simulink model "Excavator_Mevea_Bucket"  (R2026a)
settings: Solver=ode23t  StopTime=stopTime  FixedStep=1e-5  MaxStep=Ts  AbsTol=1e-3
PostLoadFcn:
  | set_param(bdroot,'IgnoredZcDiagnostic','none');
  | Excavator_Test_Scenario_Select('loadedBucketDigCycle');
  | Excavator_Mevea_params
StartFcn:
  | tStart = tic;
StopFcn:
  | elapsedSimTime = toc(tStart);
  | disp(['Elapsed Sim Time = ' num2str(elapsedSimTime)]);
model workspace: external: MAT-File ExcavatorAssemblyDataStruct.mat (data not in the file)
undefined symbols (not defined in the file or in its folder): AToBRegOrificeVector, AToTOrificeVector, BiPOrificeVector, BoomC, boomHEArea, boomREArea, boomUpMaxQ, boomValve, BToTOrificeVector, BucketC, bucketCloseMaxQ, bucketOpenMaxQ, BucketR, bucketValve, fluids, gravity, LeftBoomR, maxPumpDisp, minPumpDisp, nominalEngineSpeed, P28Assembly, PToAOrificeVector, PToBOrificeVector, pumpCmdNegRateLimit, pumpCmdPosRateLimit, RightBoomR, StickC, stickInMaxQ, stickOutMaxQ, StickR, stickValve, SwingC, swingDisplacement, swingHighSpeedThreshold, swingMaxQ, SwingR, swingSpeedQGain, swingValve, valveCmdNegRateLimit, valveCmdPosRateLimit, X, Y, Z
libraries: fl_lib x89, sm_lib x79, SimscapeFluids_lib x78, nesl_utility x57, simulink_extras x11, Excavator_Parts_Lib x6, SignalEditorBlockLib x1
(part 1 of 7)
Description:
  | Copyright 2022-2026 The MathWorks, Inc.
settings Model: VariantFading=off  Creator=gabri  LastModifiedBy=smiller
settings SolverCC: MaxConsecutiveMinStep=10  ZeroCrossAlgorithm=Adaptive  DecoupledContinuousIntegration=on  MinimalZcImpactIntegration=on
settings DataIOCC: ExternalInput=activeTestCmdsMevea  LoadExternalInput=on  SignalLoggingName=logsout_Excavator_Complete  OutputTimes=[0:Ts:stopTime]  ReturnWorkspaceOutputsName=simOut
settings DebuggingCC: IgnoredZcDiagnostic=none
settings SimscapeCC: SimscapeNominalValues="[{\"value\":\"1\",\"unit\":\"A\"},{\"value\":\"1\",\"unit\":\"bar\"},{\"value\":\"1\",\"unit\":\"cm^2\"},{\"value\":\"1\",\"unit\":\"cm^3/s\"},{\"value\":\"1\",\"unit\":\"kJ/kg\"},{\"value\":\"1\",\"unit\":\"kW\"},{\"value\":\"1\",\"unit\":\"l\"},{\"value\":\"1\",\"unit\":\"N\"},{\"value\":\"1\",\"unit\":\"N*m\"},{\"value\":\"1\",\"unit\":\"V\"}]"  SimscapeLogName=simlog_Excavator_Complete  SimscapeLogLimitData=off  SimscapeLogDataHistory=5000.0
settings DiagnosticsConfigSet: SimMechanicsUnconnectedFramePorts=none  SimMechanicsConflictingReferenceFrames=none
settings ExplorerConfigSet: InternalSimMechanicsExplorerSettings="<ExplorerConfiguration><canonicalview>default</canonicalview><AnimationSetting><BasePlaybackSpeed>1.0</BasePlaybackSpeed><PlaybackSpeedFactor>1.0</PlaybackSpeedFactor></AnimationSetting><TilePanel><TileInfo><Tiles Columns=\"1\" Count=\"1\" Rows=\"1\"><Column Weight=\"1\"/><Row Weight=\"1\"/><Tile Height=\"1\" Width=\"1\" X=\"0\" Y=\"0\"/></Tiles></TileInfo><SceneInfo><SceneViewer><BGColor><R>1</R><G>1</G><B>1</B></BGColor><Camera><DoPerspective>off</DoPerspective><Position><X>63.5460374940453718</X><Y>-11.8017502462116433</Y><Z>6.23155607724029448</Z></Position><Center><X>32.4989157916715854</X><Y>-5.03969608578851869</Y><Z>4.87768395327128346</Z></Center><Up><X>-0.0494260662251312932</X><Y>-0.0270354491512150297</Y><Z>0.998411813064479459</Z></Up><ViewLimDist>1</ViewLimDist><YLim>6.89330450435498676</YLim><XLim>8.26192051705934638</XLim></Camera></SceneViewer></SceneInfo></TilePanel><MechEditorPanel><Cameras/><GfxPanelCameraMap/><VideoCreator><PlaybackSpeedRatio>1.0</PlaybackSpeedRatio><FrameRate>30</FrameRate><VideoFormat>Motion JPEG AVI</VideoFormat><FrameSize>auto</FrameSize></VideoCreator></MechEditorPanel></ExplorerConfiguration>"

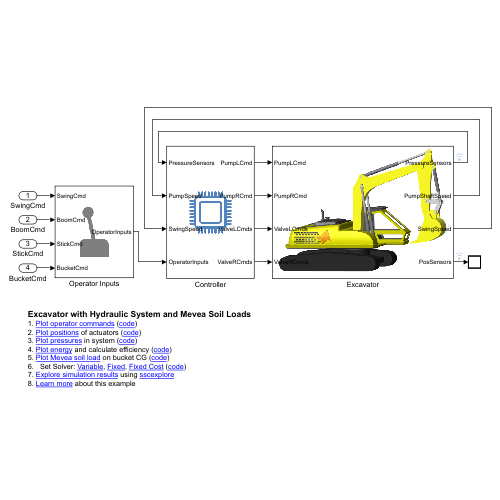
[thumbnail: Simulink's stored preview of the top-level diagram]
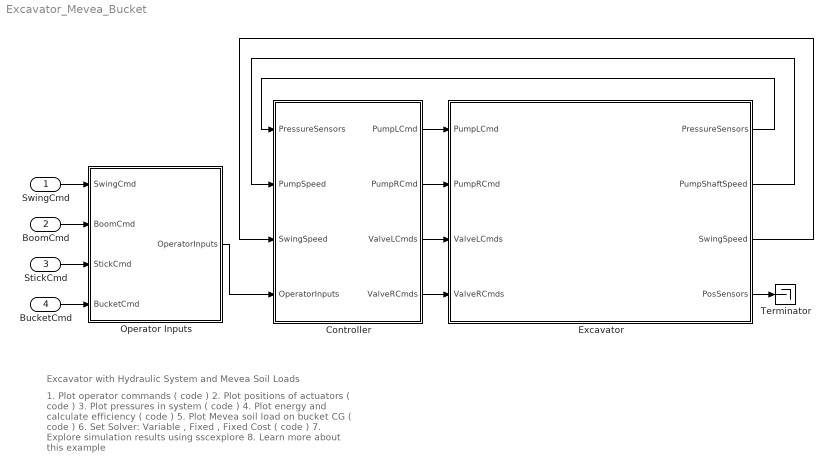
== system Excavator_Mevea_Bucket ==
  note: Excavator with Hydraulic System and Mevea Soil Loads
  note: 1. Plot operator commands ( code )
      | 2. Plot positions of actuators ( code )
      | 3. Plot pressures in system ( code )
      | 4. Plot energy and calculate efficiency ( code )
      | 5. Plot Mevea soil load on bucket CG ( code )
      | 6. Set Solver: Variable , Fixed , Fixed Cost ( code )
      | 7. Explore simulation results using sscexplore
      | 8. Learn more about this example
  SwingCmd : Inport
  BoomCmd : Inport  Port=2
  StickCmd : Inport  Port=3
  BucketCmd : Inport  Port=4
  Controller : Subsystem
      mask Display: image('Excavator_Controller_IMAGE.png')
  Excavator : Subsystem
      mask Display: image('Excavator_CAD_Full_IMAGE.png');
  Operator Inputs : Subsystem
      mask Display: image('Excavator_Operator_Inputs_IMAGE.png')
  Terminator : Terminator
  wires:
  Excavator/2(PumpShaftSpeed) -> Controller/2(PumpSpeed)
  Controller/3(ValveLCmds) -> Excavator/3(ValveLCmds)
  Operator Inputs/1(OperatorInputs) -> Controller/4(OperatorInputs)
  Excavator/1(PressureSensors) -> Controller/1(PressureSensors)
  Controller/4(ValveRCmds) -> Excavator/4(ValveRCmds)
  Controller/1(PumpLCmd) -> Excavator/1(PumpLCmd)
  Controller/2(PumpRCmd) -> Excavator/2(PumpRCmd)
  SwingCmd/1 -> Operator Inputs/1(SwingCmd)
  BoomCmd/1 -> Operator Inputs/2(BoomCmd)
  StickCmd/1 -> Operator Inputs/3(StickCmd)
  BucketCmd/1 -> Operator Inputs/4(BucketCmd)
  Excavator/3(SwingSpeed) -> Controller/3(SwingSpeed)
  Excavator/4(PosSensors) -> Terminator/1

== system Excavator_Mevea_Bucket/Controller ==
  PressureSensors : Inport
  PumpSpeed : Inport  Port=2
  SwingSpeed : Inport  Port=3
  OperatorInputs : Inport  Port=4
  Function Commander : Subsystem
  PumpLCmd : Outport
  PumpRCmd : Outport  Port=2
  ValveLCmds : Outport  Port=3
  ValveRCmds : Outport  Port=4
  wires:
  Function Commander/1(PumpLCmd) -> PumpLCmd/1
  Function Commander/3(LeftValveCmds) -> ValveLCmds/1
  Function Commander/2(PumpRCmd) -> PumpRCmd/1
  Function Commander/4(RightValveCmds) -> ValveRCmds/1
  PressureSensors/1 -> Function Commander/2(PressureSensors)
  OperatorInputs/1 -> Function Commander/1(OperatorInputs)
  PumpSpeed/1 -> Function Commander/3(PumpSpeed)
  SwingSpeed/1 -> Function Commander/4(SwingSpeed)

== system Excavator_Mevea_Bucket/Excavator ==
  PumpLCmd : Inport
  PumpRCmd : Inport  Port=2
  ValveLCmds : Inport  Port=3
  ValveRCmds : Inport  Port=4
  Engine : Subsystem
      settings: PortSchema="{\"entries\":[{\"content\":{\"sides\":[{\"content\":{\"connectorIds\":[]},\"type\":\"ConnectorPlacement.EquallySpacedRectSide\",\"uuid\":\"32d181a9-9647-459e-8a6e-f34844cbb584\"},{\"content\":{\"connectorIds\":[\"RConn1\",\"Out1\"],\"side\":\"RIGHT\"},\"type\":\"ConnectorPlacement.EquallySpacedRectSide\",\"uuid\":\"3f25e2ea-f411-44b7-ab9d-c86c977187b2\"},{\"content\":{\"connectorIds\":[],\"side\":\"TOP\"},\"type\":\"ConnectorPlacement.EquallySpacedRectSide\",\"uuid\":\"8da3c69e-7eb0-422f-a85f-a16d195e09d7\"}]},\"type\":\"ConnectorPlacement.EquallySpacedConnector\",\"uuid\":\"c91a59d7-4912-461c-aac6-1d25f9b3f709\"}],\"packageUris\":[\"http://schema.mathworks.com/mf0/Connector/R2020b\"],\"version\":\"1.0\"}"
      mask Display: image('Engine_IMAGE.png')
  Hydraulics : Subsystem
      mask Display: image('Hydraulic_System_IMAGE.png');
  Machine : Subsystem
      mask Display: image('Excavator_CAD_Full_IMAGE.png');
  PressureSensors : Outport
  PumpShaftSpeed : Outport  Port=2
  SwingSpeed : Outport  Port=3
  PosSensors : Outport  Port=4
  wires:
  Engine/1(PumpShaftSpeed) -> PumpShaftSpeed/1
  PumpLCmd/1 -> Hydraulics/1(PumpLCmd)
  PumpRCmd/1 -> Hydraulics/2(PumpRCmd)
  ValveLCmds/1 -> Hydraulics/3(ValveLCmds)
  ValveRCmds/1 -> Hydraulics/4(ValveRCmds)
  Hydraulics/1(mPr) -> PressureSensors/1
  Machine/1(SwingSpeed) -> SwingSpeed/1
  Hydraulics/2(mPos) -> PosSensors/1
  connections:
  Hydraulics/RConn1 -- Machine/LConn1
  Hydraulics/RConn2 -- Machine/LConn2
  Hydraulics/RConn3 -- Machine/LConn3
  Hydraulics/RConn4 -- Machine/LConn4
  Engine/RConn1 -- Hydraulics/LConn1

== system Excavator_Mevea_Bucket/Operator Inputs ==
  note: This Signal Editor block is here to allow for manipulation of the
      | dig cycle commands. The single function tests use the 'TestCmds'
      | scenario which is modified programatically for the function to be
      | tested when the 'TestScenarioDefinitions' script is ran.
      |
      | The inports at the top level of the model bring the commands in for
      | the simulation and are put into a bus here.
  SwingCmd : Inport
  BoomCmd : Inport  Port=2
  StickCmd : Inport  Port=3
  BucketCmd : Inport  Port=4
  OpCmdBusCreator : BusCreator  Inputs=4
  Signal Editor : SignalEditorBlockLib/Signal Editor  Commented=on  FileName=TestCommands.mat  ActiveScenario=TestCmds  ActiveSignal=SwingCmd  IsBus=off  OutputBusObjectStr=Bus: BusObject  SampleTime=0  Interpolate=off  ZeroCross=off  OutputAfterFinalValue=Setting to zero  Unit=inherit  PreserveSignalName=on  ApplySigPropsToAllScenarios=on  ApplySigPropsToAllSignals=off  SignalPropertySource=Dialog parameters
  OperatorInputs : Outport
  wires:
  OpCmdBusCreator/1 -> OperatorInputs/1
  SwingCmd/1 -> OpCmdBusCreator/1  "swingCmd"
  BoomCmd/1 -> OpCmdBusCreator/2  "boomCmd"
  StickCmd/1 -> OpCmdBusCreator/3  "stickCmd"
  BucketCmd/1 -> OpCmdBusCreator/4  "bucketCmd"

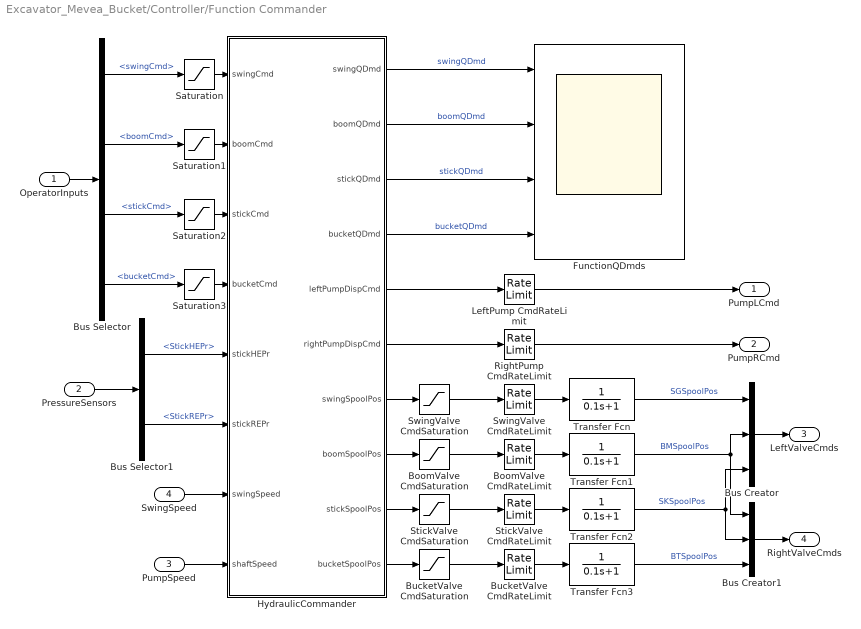
== system Excavator_Mevea_Bucket/Controller/Function Commander ==
  OperatorInputs : Inport
  PressureSensors : Inport  Port=2
  PumpSpeed : Inport  Port=3
  SwingSpeed : Inport  Port=4
  BoomValve CmdRateLimit : RateLimiter  RisingSlewLimit=valveCmdPosRateLimit  FallingSlewLimit=valveCmdNegRateLimit  SampleTimeMode=inherited
  BoomValve CmdSaturation : Saturate  UpperLimit=5  LowerLimit=-5  ZeroCross=off
  BucketValve CmdRateLimit : RateLimiter  RisingSlewLimit=valveCmdPosRateLimit  FallingSlewLimit=valveCmdNegRateLimit  SampleTimeMode=inherited
  BucketValve CmdSaturation : Saturate  UpperLimit=5  LowerLimit=-5  ZeroCross=off
  Bus Creator : BusCreator  Inputs=3
  Bus Creator1 : BusCreator  Inputs=3
  Bus Selector : BusSelector  OutputSignals=swingCmd,boomCmd,stickCmd,bucketCmd
  Bus Selector1 : BusSelector  OutputSignals=StickHEPr,StickREPr
  FunctionQDmds : Scope  NumInputPorts=4
      settings: ActiveDisplayYMinimum=-87.5  ActiveDisplayYMaximum=787.5
  HydraulicCommander : MATLAB Function  TreatAsAtomicUnit=on  mask{swingMaxQ=swingMaxQ, boomUpMaxQ=boomUpMaxQ, stickInMaxQ=stickInMaxQ, stickOutMaxQ=stickOutMaxQ, bucketOpenMaxQ=bucketOpenMaxQ, bucketCloseMaxQ=bucketCloseMaxQ, nominalShaftSpeed=nominalEngineSpeed, minPumpDisp=minPumpDisp, maxPumpDisp=maxPumpDisp, swingSpeedQGain=swingSpeedQGain, swingHighSpeedThreshold=swingHighSpeedThreshold}
      mask prompts: swingMaxQ "Swing Max Flow Rate [lpm]:"; boomUpMaxQ "Boom Up Max Flow Rate [lpm]:"; stickInMaxQ "Stick In Max Flow Rate [lpm]:"; stickOutMaxQ "Stick Out Max Flow Rate [lpm]:"; bucketOpenMaxQ "Bucket Open Max Flow Rate [lpm]:"; bucketCloseMaxQ "Bucket Close Max Flow Rate [lpm]:"; nominalShaftSpeed "Nominal Shaft Speed [rpm]:"; minPumpDisp "Minimum Pump Displacement [cc/rev]:"; maxPumpDisp "Maximum Pump Displacement [cc/rev]:"; swingSpeedQGain "Swing Flow Rate Optimization Gain:"; swingHighSpeedThreshold "Swing High Speed Threshold [rpm]:"
  LeftPump CmdRateLimit : RateLimiter  RisingSlewLimit=pumpCmdPosRateLimit  FallingSlewLimit=pumpCmdNegRateLimit  SampleTimeMode=inherited
  RightPump CmdRateLimit : RateLimiter  RisingSlewLimit=pumpCmdPosRateLimit  FallingSlewLimit=pumpCmdNegRateLimit  SampleTimeMode=inherited
  Saturation{,1..3} (4 alike) : Saturate  UpperLimit=1  LowerLimit=-1  ZeroCross=off
  StickValve CmdRateLimit : RateLimiter  RisingSlewLimit=valveCmdPosRateLimit  FallingSlewLimit=valveCmdNegRateLimit  SampleTimeMode=inherited
  StickValve CmdSaturation : Saturate  UpperLimit=5  LowerLimit=-5  ZeroCross=off
  SwingValve CmdRateLimit : RateLimiter  RisingSlewLimit=valveCmdPosRateLimit  FallingSlewLimit=valveCmdNegRateLimit  SampleTimeMode=inherited
  SwingValve CmdSaturation : Saturate  UpperLimit=5  LowerLimit=-5  ZeroCross=off
  Transfer Fcn{,1..3} (4 alike) : TransferFcn  Denominator=[0.1 1]
  PumpLCmd : Outport
  PumpRCmd : Outport  Port=2
  LeftValveCmds : Outport  Port=3
  RightValveCmds : Outport  Port=4
  wires:
  OperatorInputs/1 -> Bus Selector/1
  Bus Selector/4 -> Saturation3/1  "<bucketCmd>"
  Bus Selector/3 -> Saturation2/1  "<stickCmd>"
  Bus Selector/2 -> Saturation1/1  "<boomCmd>"
  Bus Selector/1 -> Saturation/1  "<swingCmd>"
  PumpSpeed/1 -> HydraulicCommander/8(shaftSpeed)
  PressureSensors/1 -> Bus Selector1/1
  Bus Selector1/1 -> HydraulicCommander/5(stickHEPr)  "<StickHEPr>"
  Bus Selector1/2 -> HydraulicCommander/6(stickREPr)  "<StickREPr>"
  Bus Creator/1 -> LeftValveCmds/1
  Bus Creator1/1 -> RightValveCmds/1
  HydraulicCommander/1(swingQDmd) -> FunctionQDmds/1  "swingQDmd"
  HydraulicCommander/2(boomQDmd) -> FunctionQDmds/2  "boomQDmd"
  HydraulicCommander/3(stickQDmd) -> FunctionQDmds/3  "stickQDmd"
  HydraulicCommander/4(bucketQDmd) -> FunctionQDmds/4  "bucketQDmd"
  Transfer Fcn1/1 -> Bus Creator1/1, Bus Creator/2  "BMSpoolPos"
  Transfer Fcn/1 -> Bus Creator/1  "SGSpoolPos"
  Transfer Fcn2/1 -> Bus Creator1/2, Bus Creator/3  "SKSpoolPos"
  Transfer Fcn3/1 -> Bus Creator1/3  "BTSpoolPos"
  LeftPump CmdRateLimit/1 -> PumpLCmd/1
  RightPump CmdRateLimit/1 -> PumpRCmd/1
  Saturation/1 -> HydraulicCommander/1(swingCmd)
  Saturation1/1 -> HydraulicCommander/2(boomCmd)
  Saturation2/1 -> HydraulicCommander/3(stickCmd)
  Saturation3/1 -> HydraulicCommander/4(bucketCmd)
  SwingSpeed/1 -> HydraulicCommander/7(swingSpeed)
  SwingValve CmdSaturation/1 -> SwingValve CmdRateLimit/1
  BoomValve CmdSaturation/1 -> BoomValve CmdRateLimit/1
  StickValve CmdSaturation/1 -> StickValve CmdRateLimit/1
  BucketValve CmdSaturation/1 -> BucketValve CmdRateLimit/1
  HydraulicCommander/5(leftPumpDispCmd) -> LeftPump CmdRateLimit/1
  HydraulicCommander/6(rightPumpDispCmd) -> RightPump CmdRateLimit/1
  HydraulicCommander/7(swingSpoolPos) -> SwingValve CmdSaturation/1
  HydraulicCommander/8(boomSpoolPos) -> BoomValve CmdSaturation/1
  HydraulicCommander/9(stickSpoolPos) -> StickValve CmdSaturation/1
  HydraulicCommander/10(bucketSpoolPos) -> BucketValve CmdSaturation/1
  SwingValve CmdRateLimit/1 -> Transfer Fcn/1
  BoomValve CmdRateLimit/1 -> Transfer Fcn1/1
  StickValve CmdRateLimit/1 -> Transfer Fcn2/1
  BucketValve CmdRateLimit/1 -> Transfer Fcn3/1

== system Excavator_Mevea_Bucket/Excavator/Engine ==
  Engine : fl_lib/Mechanical/Mechanical Sources/Ideal Angular Velocity Source
  EngineRotationalRef : fl_lib/Mechanical/Rotational Elements/Mechanical Rotational Reference
  Ideal Rotational Motion Sensor : fl_lib/Mechanical/Mechanical Sensors/Ideal Rotational Motion Sensor  reference=foundation.enum.MeasurementReference.difference  acceleration_port=false  velocity_port=true  position_port=true  wrap_angle=simscape.enum.onoff.off  offset=0 rad
  PS Constant : fl_lib/Physical Signals/Sources/PS Constant  constant=1500 rpm
  PS-Simulink Converter : nesl_utility/PS-Simulink Converter  PhysicalDomain=network_engine_domain  SubClassName=ps_output  LeftPortType=input  RightPortType=output  PseudoPeriodic=off  Frequencies=[]  VectorFormat=1-D array  Unit=rpm  AffineConversion=off
  PS-Simulink Converter3 : nesl_utility/PS-Simulink Converter  PhysicalDomain=network_engine_domain  SubClassName=ps_output  LeftPortType=input  RightPortType=output  PseudoPeriodic=off  Frequencies=[]  VectorFormat=1-D array  Unit=rad  AffineConversion=off
  Terminator : Terminator
  Transfer Fcn (with initial outputs) : simulink_extras/Additional Linear/Transfer Fcn (with initial outputs)  N=[1]  D="[0.01  1]"  Y0=1500  U0=1500
  Shaft : PMIOPort  Side=Right
  PumpShaftSpeed : Outport
  wires:
  PS-Simulink Converter/1 -> Transfer Fcn (with initial outputs)/1
  PS-Simulink Converter3/1 -> Terminator/1
  Transfer Fcn (with initial outputs)/1 -> PumpShaftSpeed/1
  connections:
  PS Constant/RConn1 -- Engine/RConn1
  Engine/RConn2 -- Ideal Rotational Motion Sensor/RConn1 -- EngineRotationalRef/LConn1
  Shaft/RConn1 -- Ideal Rotational Motion Sensor/LConn1 -- Engine/LConn1
  PS-Simulink Converter3/LConn1 -- Ideal Rotational Motion Sensor/RConn3
  Ideal Rotational Motion Sensor/RConn2 -- PS-Simulink Converter/LConn1

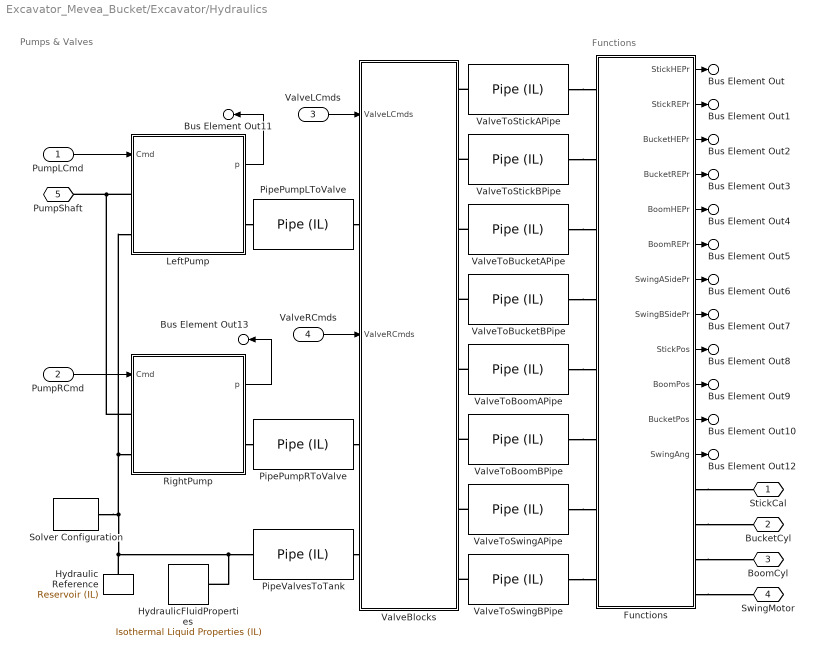
== system Excavator_Mevea_Bucket/Excavator/Hydraulics ==
  note: Functions
  note: Pumps & Valves
  PumpLCmd : Inport
  PumpRCmd : Inport  Port=2
  ValveLCmds : Inport  Port=3
  ValveRCmds : Inport  Port=4
  Functions : Subsystem
      mask Display: image('Hydraulic_Actuators_All_IMAGE.png');
  Hydraulic Reference : fl_lib/Isothermal Liquid/Elements/Reservoir (IL)  pressure_input=false  pressure_spec=foundation.enum.pressure_spec.atmospheric  reservoir_pressure=0.101325 MPa
  HydraulicFluidProperties : fl_lib/Isothermal Liquid/Utilities/Isothermal Liquid Properties (IL)  rho_L_atm=870 kg/m^3  bulk_modulus_model=foundation.enum.bulk_modulus_model.const  beta_gain=6  beta_L_atm=1.45e9 Pa  nu_atm=46 mm^2/s  p_atm=0.101325 MPa  p_min=0.1 Pa  properties_range_check=simscape.enum.assert.action.error  air_fraction=0.005  polytropic_index=1.0  rho_g_atm=1.225 kg/m^3  air_dissolution_model=simscape.enum.onoff.off  p_crit=3 MPa
  LeftPump : Subsystem
      mask Display: image('Hydraulic_Pump_IMAGE.png')
  PipePumpLToValve : fl_lib/Isothermal Liquid/Elements/Pipe (IL)  length=pipeLength mm  area=pipeCrossSectArea mm^2  Dh=pipeHydraulicDiam mm  length_add=1 m  roughness=15e-6 m  Re_lam=2000  Re_tur=4000  shape_factor=64  dynamic_compressibility=simscape.enum.onoff.off  inertia=simscape.enum.onoff.off  p0=0.101325 MPa  mdot0=0 kg/s
  PipePumpRToValve : fl_lib/Isothermal Liquid/Elements/Pipe (IL)  length=pipeLength mm  area=pipeCrossSectArea mm^2  Dh=pipeHydraulicDiam mm  length_add=1 m  roughness=15e-6 m  Re_lam=2000  Re_tur=4000  shape_factor=64  dynamic_compressibility=simscape.enum.onoff.off  inertia=simscape.enum.onoff.off  p0=0.101325 MPa  mdot0=0 kg/s
  PipeValvesToTank : fl_lib/Isothermal Liquid/Elements/Pipe (IL)  length=pipeLength mm  area=pipeCrossSectArea mm^2  Dh=pipeHydraulicDiam mm  length_add=1 m  roughness=15e-6 m  Re_lam=2000  Re_tur=4000  shape_factor=64  dynamic_compressibility=simscape.enum.onoff.off  inertia=simscape.enum.onoff.off  p0=0.101325 MPa  mdot0=0 kg/s
  RightPump : Subsystem
      mask Display: image('Hydraulic_Pump_IMAGE.png')
  Solver Configuration : nesl_utility/Solver Configuration  PhysicalDomain=network_engine_domain  SubClassName=solver  LeftPortType=input  RightPortType=generic  Tones=[]  Harmonics=[]  SimulateNoise=off  Profile=off  UseLocalSampling=off  EnableSwitchedLinearOptims=on  FrequencyDomain=off  UseCCode=off  RelTol=0.001  AbsTol=1e-06  MinStep=1e-09  ToWorkspace=off  RevertToSquareIcSolve=off  NumHomotopyIterations=100  PhasorMode=off  PhasorModeNumHarmonics=1  ConsistencySolver=NEWTON_FTOL  CanonicalOrdering=UNORDERED  OptimizeIntermediates=UNOPTIMIZED  IndexReductionMethod=DerivativeReplacement  DoDC=off  ResidualTolerance=1e-09  ConsistencyTolSource=GLOBAL  ConsistencyAbsTol=0.001  ConsistencyRelTol=0.001  ConsistencyTolFactor=0.001  UseLocalSolver=off  LocalSolverChoice=NE_BACKWARD_EULER_ADVANCER  ResolveIndetEquations=on  FunctionEvalNumThread=1  LocalSolverSampleTime=0.001  DoFixedCost=off  MaxNonlinIter=3  MaxModeIter=2  ComputeImpulses=off  ImpulseIterations=2  LinearAlgebra=auto  LinearAlgebraNumThread=0  EquationFormulation=NE_TIME_EF  DelaysMemoryBudget=1024  AutomaticFiltering=on  FilteringTimeConstant=0.001  PartitionStorageMethod=AS_NEEDED  PartitionMemoryBudget=1024  PartitionMethod=ROBUST  MultibodyUseLocalSolver=off  MultibodyLocalSolverChoice=ODE1  MultibodyLocalSolverSampleTime=0.001
  ValveBlocks : Subsystem
      settings: PortSchema="{\"entries\":[{\"content\":{\"sides\":[{\"content\":{\"connectorIds\":[\"In1\",\"LConn1\",\"In2\",\"LConn2\",\"LConn3\"]},\"type\":\"ConnectorPlacement.EquallySpacedRectSide\",\"uuid\":\"b3bc2bda-0212-4e11-9874-ac6e4fe9b6a3\"},{\"content\":{\"connectorIds\":[\"RConn1\",\"RConn2\",\"RConn3\",\"RConn4\",\"RConn5\",\"RConn6\",\"RConn7\",\"RConn8\"],\"side\":\"RIGHT\"},\"type\":\"ConnectorPlacement.EquallySpacedRectSide\",\"uuid\":\"c9983e91-7586-4f39-92a2-b2598f03e211\"},{\"content\":{\"connectorIds\":[],\"side\":\"TOP\"},\"type\":\"ConnectorPlacement.EquallySpacedRectSide\",\"uuid\":\"d3f67102-423e-42f5-ac92-8a3282aefd24\"}]},\"type\":\"ConnectorPlacement.EquallySpacedConnector\",\"uuid\":\"bd5efcea-2b0a-45c5-b20e-e10c208a7bb5\"}],\"packageUris\":[\"http://schema.mathworks.com/mf0/Connector/R2020b\"],\"version\":\"1.0\"}"
      mask Display: image('Valve_Block_All_IMAGE.png')
  ValveToBoomAPipe : fl_lib/Isothermal Liquid/Elements/Pipe (IL)  length=pipeLength mm  area=pipeCrossSectArea mm^2  Dh=pipeHydraulicDiam mm  length_add=1 m  roughness=15e-6 m  Re_lam=2000  Re_tur=4000  shape_factor=64  dynamic_compressibility=simscape.enum.onoff.off  inertia=simscape.enum.onoff.off  p0=0.101325 MPa  mdot0=0 kg/s
  ValveToBoomBPipe : fl_lib/Isothermal Liquid/Elements/Pipe (IL)  length=pipeLength mm  area=pipeCrossSectArea mm^2  Dh=pipeHydraulicDiam mm  length_add=1 m  roughness=15e-6 m  Re_lam=2000  Re_tur=4000  shape_factor=64  dynamic_compressibility=simscape.enum.onoff.off  inertia=simscape.enum.onoff.off  p0=0.101325 MPa  mdot0=0 kg/s
  ValveToBucketAPipe : fl_lib/Isothermal Liquid/Elements/Pipe (IL)  length=pipeLength mm  area=pipeCrossSectArea mm^2  Dh=pipeHydraulicDiam mm  length_add=1 m  roughness=15e-6 m  Re_lam=2000  Re_tur=4000  shape_factor=64  dynamic_compressibility=simscape.enum.onoff.off  inertia=simscape.enum.onoff.off  p0=0.101325 MPa  mdot0=0 kg/s
  ValveToBucketBPipe : fl_lib/Isothermal Liquid/Elements/Pipe (IL)  length=pipeLength mm  area=pipeCrossSectArea mm^2  Dh=pipeHydraulicDiam mm  length_add=1 m  roughness=15e-6 m  Re_lam=2000  Re_tur=4000  shape_factor=64  dynamic_compressibility=simscape.enum.onoff.off  inertia=simscape.enum.onoff.off  p0=0.101325 MPa  mdot0=0 kg/s
  ValveToStickAPipe : fl_lib/Isothermal Liquid/Elements/Pipe (IL)  length=pipeLength mm  area=pipeCrossSectArea mm^2  Dh=pipeHydraulicDiam mm  length_add=1 m  roughness=15e-6 m  Re_lam=2000  Re_tur=4000  shape_factor=64  dynamic_compressibility=simscape.enum.onoff.off  inertia=simscape.enum.onoff.off  p0=0.101325 MPa  mdot0=0 kg/s
  ValveToStickBPipe : fl_lib/Isothermal Liquid/Elements/Pipe (IL)  length=pipeLength mm  area=pipeCrossSectArea mm^2  Dh=pipeHydraulicDiam mm  length_add=1 m  roughness=15e-6 m  Re_lam=2000  Re_tur=4000  shape_factor=64  dynamic_compressibility=simscape.enum.onoff.off  inertia=simscape.enum.onoff.off  p0=0.101325 MPa  mdot0=0 kg/s
  ValveToSwingAPipe : fl_lib/Isothermal Liquid/Elements/Pipe (IL)  length=pipeLength mm  area=pipeCrossSectArea mm^2  Dh=pipeHydraulicDiam mm  length_add=1 m  roughness=15e-6 m  Re_lam=2000  Re_tur=4000  shape_factor=64  dynamic_compressibility=false  inertia=simscape.enum.onoff.off  p0=initSwingAPr MPa  mdot0=0 kg/s
  ValveToSwingBPipe : fl_lib/Isothermal Liquid/Elements/Pipe (IL)  length=pipeLength mm  area=pipeCrossSectArea mm^2  Dh=pipeHydraulicDiam mm  length_add=1 m  roughness=15e-6 m  Re_lam=2000  Re_tur=4000  shape_factor=64  dynamic_compressibility=false  inertia=simscape.enum.onoff.off  p0=initSwingAPr MPa  mdot0=0 kg/s
  StickCal : PMIOPort  Side=Right
  BucketCyl : PMIOPort  Port=2  Side=Right
  BoomCyl : PMIOPort  Port=3  Side=Right
  SwingMotor : PMIOPort  Port=4  Side=Right
  PumpShaft : PMIOPort  Port=5  Side=Left
  Bus Element Out : Outport  PortName=mPr  Element=StickHEPr
  Bus Element Out1 : Outport  PortName=mPr  Element=StickREPr
  Bus Element Out2 : Outport  PortName=mPr  Element=BucketHEPr
  Bus Element Out3 : Outport  PortName=mPr  Element=BucketREPr
  Bus Element Out4 : Outport  PortName=mPr  Element=BoomHEPr
  Bus Element Out5 : Outport  PortName=mPr  Element=BoomREPr
  Bus Element Out6 : Outport  PortName=mPr  Element=SwingASidePr
  Bus Element Out7 : Outport  PortName=mPr  Element=SwingBSidePr
  Bus Element Out11 : Outport  PortName=mPr  Element=LeftPumpPr
  Bus Element Out13 : Outport  PortName=mPr  Element=RightPumpPr
  Bus Element Out12 : Outport  Port=2  PortName=mPos  Element=SwingAng
  Bus Element Out10 : Outport  Port=2  PortName=mPos  Element=BucketPos
  Bus Element Out9 : Outport  Port=2  PortName=mPos  Element=BoomPos
  Bus Element Out8 : Outport  Port=2  PortName=mPos  Element=StickPos
  wires:
  RightPump/1(p) -> Bus Element Out13/1
  PumpLCmd/1 -> LeftPump/1(Cmd)
  LeftPump/1(p) -> Bus Element Out11/1
  ValveRCmds/1 -> ValveBlocks/2(ValveRCmds)
  ValveLCmds/1 -> ValveBlocks/1(ValveLCmds)
  Functions/1(StickHEPr) -> Bus Element Out/1
  Functions/3(BucketHEPr) -> Bus Element Out2/1
  Functions/5(BoomHEPr) -> Bus Element Out4/1
  Functions/7(SwingASidePr) -> Bus Element Out6/1
  Functions/8(SwingBSidePr) -> Bus Element Out7/1
  Functions/6(BoomREPr) -> Bus Element Out5/1
  Functions/4(BucketREPr) -> Bus Element Out3/1
  Functions/2(StickREPr) -> Bus Element Out1/1
  PumpRCmd/1 -> RightPump/1(Cmd)
  Functions/9(StickPos) -> Bus Element Out8/1
  Functions/10(BoomPos) -> Bus Element Out9/1
  Functions/11(BucketPos) -> Bus Element Out10/1
  Functions/12(SwingAng) -> Bus Element Out12/1
  connections:
  LeftPump/LConn1 -- PumpShaft/RConn1 -- RightPump/LConn1
  LeftPump/RConn1 -- PipePumpLToValve/LConn1
  RightPump/RConn1 -- PipePumpRToValve/LConn1
  Functions/RConn1 -- StickCal/RConn1
  Functions/RConn2 -- BucketCyl/RConn1
  Functions/RConn3 -- BoomCyl/RConn1
  Functions/RConn4 -- SwingMotor/RConn1
  PipePumpLToValve/RConn1 -- ValveBlocks/LConn1
  PipePumpRToValve/RConn1 -- ValveBlocks/LConn2
  ValveToStickAPipe/LConn1 -- ValveBlocks/RConn1
  ValveToStickBPipe/LConn1 -- ValveBlocks/RConn2
  ValveToBucketAPipe/LConn1 -- ValveBlocks/RConn3
  ValveToBucketBPipe/LConn1 -- ValveBlocks/RConn4
  ValveToBoomAPipe/LConn1 -- ValveBlocks/RConn5
  ValveToBoomBPipe/LConn1 -- ValveBlocks/RConn6
  ValveToSwingAPipe/LConn1 -- ValveBlocks/RConn7
  ValveToSwingBPipe/LConn1 -- ValveBlocks/RConn8
  ValveToSwingBPipe/RConn1 -- Functions/LConn8
  ValveToSwingAPipe/RConn1 -- Functions/LConn7
  ValveToBoomBPipe/RConn1 -- Functions/LConn6
  ValveToBoomAPipe/RConn1 -- Functions/LConn5
  ValveToBucketBPipe/RConn1 -- Functions/LConn4
  ValveToBucketAPipe/RConn1 -- Functions/LConn3
  ValveToStickBPipe/RConn1 -- Functions/LConn2
  ValveToStickAPipe/RConn1 -- Functions/LConn1
  RightPump/LConn2 -- Hydraulic Reference/LConn1 -- HydraulicFluidProperties/RConn1 -- PipeValvesToTank/RConn1 -- Solver Configuration/RConn1 -- LeftPump/LConn2
  PipeValvesToTank/LConn1 -- ValveBlocks/LConn3

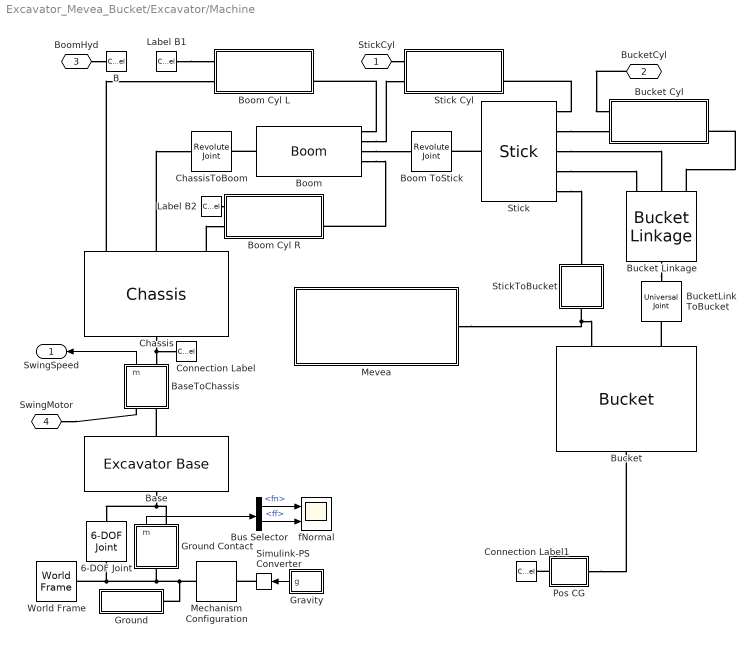
== system Excavator_Mevea_Bucket/Excavator/Machine ==
  6-DOF Joint : sm_lib/Joints/6-DOF Joint  JointMode=Normal  CompositeWrenchDir=FollowerOnBase  CompositeWrenchFrame=BaseFrame  SenseConstraintForce=off  SenseConstraintTorque=off  SenseTotalForce=off  SenseTotalTorque=off  PxPositionTargetSpecify=off  PxPositionTargetPriority=High  PxPositionTargetValue=0  PxPositionTargetValueUnits=m  PxVelocityTargetSpecify=off  PxVelocityTargetPriority=High  PxVelocityTargetValue=0  PxVelocityTargetValueUnits=m/s  PxEquilibriumPosition=0  PxEquilibriumPositionUnits=m  PxSpringStiffness=0  PxSpringStiffnessUnits=N/m  PxDampingCoefficient=0  PxDampingCoefficientUnits=N/(m/s)  PxLowerLimitSpecify=off  PxLowerLimitBound=-1  PxLowerLimitBoundUnits=m  PxLowerLimitStiffness=1e6  PxLowerLimitStiffnessUnits=N/m  PxLowerLimitDamping=1e3  PxLowerLimitDampingUnits=N/(m/s)  PxLowerLimitTransitionRegionWidth=1e-4  PxLowerLimitTransitionRegionWidthUnits=m  PxUpperLimitSpecify=off  PxUpperLimitBound=1  PxUpperLimitBoundUnits=m  PxUpperLimitStiffness=1e6  PxUpperLimitStiffnessUnits=N/m  PxUpperLimitDamping=1e3  PxUpperLimitDampingUnits=N/(m/s)  PxUpperLimitTransitionRegionWidth=1e-4  PxUpperLimitTransitionRegionWidthUnits=m  PxTorqueActuationMode=NoTorque  PxMotionActuationMode=ComputedMotion  PxSensePosition=off  PxSenseVelocity=off  PxSenseAcceleration=off  PxSenseTorqueForce=off  PxSenseLowerLimitTorqueForce=off  PxSenseUpperLimitTorqueForce=off  PyPositionTargetSpecify=off  PyPositionTargetPriority=High  PyPositionTargetValue=0  PyPositionTargetValueUnits=m  PyVelocityTargetSpecify=off  PyVelocityTargetPriority=High  PyVelocityTargetValue=0  PyVelocityTargetValueUnits=m/s  PyEquilibriumPosition=0  PyEquilibriumPositionUnits=m  PySpringStiffness=0  PySpringStiffnessUnits=N/m  PyDampingCoefficient=0  PyDampingCoefficientUnits=N/(m/s)  PyLowerLimitSpecify=off  PyLowerLimitBound=-1  PyLowerLimitBoundUnits=m  PyLowerLimitStiffness=1e6  PyLowerLimitStiffnessUnits=N/m  PyLowerLimitDamping=1e3  PyLowerLimitDampingUnits=N/(m/s)  PyLowerLimitTransitionRegionWidth=1e-4  PyLowerLimitTransitionRegionWidthUnits=m  PyUpperLimitSpecify=off  PyUpperLimitBound=1  PyUpperLimitBoundUnits=m  PyUpperLimitStiffness=1e6  PyUpperLimitStiffnessUnits=N/m  PyUpperLimitDamping=1e3  PyUpperLimitDampingUnits=N/(m/s)  PyUpperLimitTransitionRegionWidth=1e-4  PyUpperLimitTransitionRegionWidthUnits=m  PyTorqueActuationMode=NoTorque  PyMotionActuationMode=ComputedMotion  PySensePosition=off  PySenseVelocity=off  PySenseAcceleration=off  PySenseTorqueForce=off  PySenseLowerLimitTorqueForce=off  PySenseUpperLimitTorqueForce=off  PzPositionTargetSpecify=off  PzPositionTargetPriority=High  PzPositionTargetValue=0  PzPositionTargetValueUnits=m  PzVelocityTargetSpecify=off  PzVelocityTargetPriority=High  PzVelocityTargetValue=0  PzVelocityTargetValueUnits=m/s  PzEquilibriumPosition=0  PzEquilibriumPositionUnits=m  PzSpringStiffness=0  PzSpringStiffnessUnits=N/m  PzDampingCoefficient=0  PzDampingCoefficientUnits=N/(m/s)  PzLowerLimitSpecify=off  PzLowerLimitBound=-1  PzLowerLimitBoundUnits=m  PzLowerLimitStiffness=1e6  PzLowerLimitStiffnessUnits=N/m  PzLowerLimitDamping=1e3  PzLowerLimitDampingUnits=N/(m/s)  PzLowerLimitTransitionRegionWidth=1e-4  PzLowerLimitTransitionRegionWidthUnits=m  PzUpperLimitSpecify=off  PzUpperLimitBound=1  PzUpperLimitBoundUnits=m  PzUpperLimitStiffness=1e6  PzUpperLimitStiffnessUnits=N/m  PzUpperLimitDamping=1e3  PzUpperLimitDampingUnits=N/(m/s)  PzUpperLimitTransitionRegionWidth=1e-4  PzUpperLimitTransitionRegionWidthUnits=m  PzTorqueActuationMode=NoTorque  PzMotionActuationMode=ComputedMotion  PzSensePosition=off  PzSenseVelocity=off  PzSenseAcceleration=off  PzSenseTorqueForce=off  PzSenseLowerLimitTorqueForce=off  PzSenseUpperLimitTorqueForce=off  SphPositionTargetSpecify=off  SphPositionTargetPriority=High  SphPositionTargetRotationMethod=None  SphPositionTargetFollAlignAxisA=+X  SphPositionTargetBaseAlignAxisA=+Y  SphPositionTargetFollAlignAxisB=+Y  SphPositionTargetBaseAlignAxisB=+Z  SphPositionTargetRotationStandardAxis=+Z  SphPositionTargetRotationAngle=0.0  SphPositionTargetRotationAngleUnits=deg  SphPositionTargetRotationArbitraryAxis=[0 0 1]  SphPositionTargetRotationSequenceAxes=FollowerAxes  SphPositionTargetRotationSequence=XYX  SphPositionTargetRotationSequenceAngles=[0 0 0]  SphPositionTargetRotationSequenceAnglesUnits=deg  SphPositionTargetRotationMatrix=[1 0 0; 0 1 0; 0 0 1]  SphPositionTargetQuaternion=[1 0 0 0]  SphVelocityTargetSpecify=off  SphVelocityTargetPriority=High  SphVelocityTargetValue=[0 0 0]  SphVelocityTargetValueUnits=deg/s  SphVelocityTargetInFollowerFrame=on  SphEqPosRotationMethod=None  SphEqPosFollAlignAxisA=+X  SphEqPosBaseAlignAxisA=+Y  SphEqPosFollAlignAxisB=+Y  SphEqPosBaseAlignAxisB=+Z  SphEqPosRotationStandardAxis=+Z  SphEqPosRotationAngle=0.0  SphEqPosRotationAngleUnits=deg  SphEqPosRotationArbitraryAxis=[0 0 1]  SphEqPosRotationSequenceAxes=FollowerAxes  SphEqPosRotationSequence=XYX  SphEqPosRotationSequenceAngles=[0 0 0]  SphEqPosRotationSequenceAnglesUnits=deg  SphEqPosRotationMatrix=[1 0 0; 0 1 0; 0 0 1]  SphEqPosQuaternion=[1 0 0 0]  SphSpringStiffness=0  SphSpringStiffnessUnits=N*m/deg  SphDampingCoefficient=0  SphDampingCoefficientUnits=N*m/(deg/s)  SphLowerLimitSpecify=off  SphLowerLimitBound=15  SphLowerLimitBoundUnits=deg  SphLowerLimitStiffness=1e4  SphLowerLimitStiffnessUnits=N*m/deg  SphLowerLimitDamping=10  SphLowerLimitDampingUnits=N*m/(deg/s)  SphLowerLimitTransitionRegionWidth=0.1  SphLowerLimitTransitionRegionWidthUnits=deg  SphUpperLimitSpecify=off  SphUpperLimitBound=45  SphUpperLimitBoundUnits=deg  SphUpperLimitStiffness=1e4  SphUpperLimitStiffnessUnits=N*m/deg  SphUpperLimitDamping=10  SphUpperLimitDampingUnits=N*m/(deg/s)  SphUpperLimitTransitionRegionWidth=0.1  SphUpperLimitTransitionRegionWidthUnits=deg  SphTorqueActuationMode=NoTorque  SphActuateTorqueX=off  SphActuateTorqueY=off  SphActuateTorqueZ=off  SphActuateTorque=off  SphActuationFrame=BaseFrame  SphSensePosition=off  SphSenseVelocityX=off  SphSenseVelocityY=off  SphSenseVelocityZ=off  SphSenseVelocity=off  SphSenseAccelerationX=off  SphSenseAccelerationY=off  SphSenseAccelerationZ=off  SphSenseAcceleration=off  SphSenseLowerLimitTorqueMag=off  SphSenseUpperLimitTorqueMag=off  SphSensingFrame=BaseFrame
  B : ConnectionLabel  Label=B
  Base : Excavator_Parts_Lib/Excavator Base  Tag=AAA55596-1DB0-4345-9724-6685E48489E2
  BaseToChassis : Subsystem  Tag=1fdcb50d-bed1-4557-9df5-71c57fded59e
      mask Display: image('Excavator_Revolute_IMAGE.png')
  Boom : Excavator_Parts_Lib/Boom  Tag=FF941BC7-23B6-8A4E-AE2C-D7583C913694  opc=1  part_clr=excv_data.arm.clr
  Boom ToStick : sm_lib/Joints/Revolute Joint  JointMode=Normal  CompositeWrenchDir=FollowerOnBase  CompositeWrenchFrame=BaseFrame  SenseConstraintForce=off  SenseConstraintTorque=off  SenseTotalForce=off  SenseTotalTorque=off  PositionTargetSpecify=on  PositionTargetPriority=Low  PositionTargetValue=initBoomToStickRevPos  PositionTargetValueUnits=deg  VelocityTargetSpecify=off  VelocityTargetPriority=High  VelocityTargetValue=0  VelocityTargetValueUnits=deg/s  EquilibriumPosition=0  EquilibriumPositionUnits=deg  SpringStiffness=0  SpringStiffnessUnits=N*m/deg  DampingCoefficient=0  DampingCoefficientUnits=N*m/(deg/s)  LowerLimitSpecify=off  LowerLimitBound=-90  LowerLimitBoundUnits=deg  LowerLimitStiffness=1e4  LowerLimitStiffnessUnits=N*m/deg  LowerLimitDamping=10  LowerLimitDampingUnits=N*m/(deg/s)  LowerLimitTransitionRegionWidth=0.1  LowerLimitTransitionRegionWidthUnits=deg  UpperLimitSpecify=off  UpperLimitBound=90  UpperLimitBoundUnits=deg  UpperLimitStiffness=1e4  UpperLimitStiffnessUnits=N*m/deg  UpperLimitDamping=10  UpperLimitDampingUnits=N*m/(deg/s)  UpperLimitTransitionRegionWidth=0.1  UpperLimitTransitionRegionWidthUnits=deg  TorqueActuationMode=NoTorque  MotionActuationMode=ComputedMotion  SensePosition=off  SenseVelocity=off  SenseAcceleration=off  SenseTorqueForce=off  SenseLowerLimitTorqueForce=off  SenseUpperLimitTorqueForce=off
  Boom Cyl L : Subsystem
      mask Display: image('Excavator_Cylinder_Actuate_IMAGE.png')
  Boom Cyl R : Subsystem
      mask Display: image('Excavator_Cylinder_Actuate_IMAGE.png')
  Bucket : Excavator_Parts_Lib/Bucket  Tag=FF47B028-216B-7042-A7FD-934F60E6CEA6  opc=1  part_clr=excv_data.arm.clr
  Bucket Linkage : Excavator_Parts_Lib/Bucket Linkage
  Bucket Cyl : Subsystem
      mask Display: image('Excavator_Cylinder_Actuate_IMAGE.png')
  BucketLink ToBucket : sm_lib/Joints/Universal Joint  JointMode=Normal  CompositeWrenchDir=FollowerOnBase  CompositeWrenchFrame=BaseFrame  SenseConstraintForce=off  SenseConstraintTorque=off  SenseTotalForce=off  SenseTotalTorque=off  RxPositionTargetSpecify=off  RxPositionTargetPriority=Low  RxPositionTargetValue=0  RxPositionTargetValueUnits=deg  RxVelocityTargetSpecify=off  RxVelocityTargetPriority=High  RxVelocityTargetValue=0  RxVelocityTargetValueUnits=deg/s  RxEquilibriumPosition=0  RxEquilibriumPositionUnits=deg  RxSpringStiffness=0  RxSpringStiffnessUnits=N*m/deg  RxDampingCoefficient=0  RxDampingCoefficientUnits=N*m/(deg/s)  RxLowerLimitSpecify=off  RxLowerLimitBound=-90  RxLowerLimitBoundUnits=deg  RxLowerLimitStiffness=1e4  RxLowerLimitStiffnessUnits=N*m/deg  RxLowerLimitDamping=10  RxLowerLimitDampingUnits=N*m/(deg/s)  RxLowerLimitTransitionRegionWidth=0.1  RxLowerLimitTransitionRegionWidthUnits=deg  RxUpperLimitSpecify=off  RxUpperLimitBound=90  RxUpperLimitBoundUnits=deg  RxUpperLimitStiffness=1e4  RxUpperLimitStiffnessUnits=N*m/deg  RxUpperLimitDamping=10  RxUpperLimitDampingUnits=N*m/(deg/s)  RxUpperLimitTransitionRegionWidth=0.1  RxUpperLimitTransitionRegionWidthUnits=deg  RxTorqueActuationMode=NoTorque  RxMotionActuationMode=ComputedMotion  RxSensePosition=off  RxSenseVelocity=off  RxSenseAcceleration=off  RxSenseTorqueForce=off  RxSenseLowerLimitTorqueForce=off  RxSenseUpperLimitTorqueForce=off  RyPositionTargetSpecify=off  RyPositionTargetPriority=Low  RyPositionTargetValue=0  RyPositionTargetValueUnits=deg  RyVelocityTargetSpecify=off  RyVelocityTargetPriority=High  RyVelocityTargetValue=0  RyVelocityTargetValueUnits=deg/s  RyEquilibriumPosition=0  RyEquilibriumPositionUnits=deg  RySpringStiffness=0  RySpringStiffnessUnits=N*m/deg  RyDampingCoefficient=0  RyDampingCoefficientUnits=N*m/(deg/s)  RyLowerLimitSpecify=off  RyLowerLimitBound=-90  RyLowerLimitBoundUnits=deg  RyLowerLimitStiffness=1e4  RyLowerLimitStiffnessUnits=N*m/deg  RyLowerLimitDamping=10  RyLowerLimitDampingUnits=N*m/(deg/s)  RyLowerLimitTransitionRegionWidth=0.1  RyLowerLimitTransitionRegionWidthUnits=deg  RyUpperLimitSpecify=off  RyUpperLimitBound=90  RyUpperLimitBoundUnits=deg  RyUpperLimitStiffness=1e4  RyUpperLimitStiffnessUnits=N*m/deg  RyUpperLimitDamping=10  RyUpperLimitDampingUnits=N*m/(deg/s)  RyUpperLimitTransitionRegionWidth=0.1  RyUpperLimitTransitionRegionWidthUnits=deg  RyTorqueActuationMode=NoTorque  RyMotionActuationMode=ComputedMotion  RySensePosition=off  RySenseVelocity=off  RySenseAcceleration=off  RySenseTorqueForce=off  RySenseLowerLimitTorqueForce=off  RySenseUpperLimitTorqueForce=off
  Bus Selector : BusSelector  OutputSignals=fn,ff
  Chassis : Excavator_Parts_Lib/Chassis  Tag=19F311DB-9E7A-8F4D-82CB-D8DCD5D4899B  opc=1
  ChassisToBoom : sm_lib/Joints/Revolute Joint  JointMode=Normal  CompositeWrenchDir=FollowerOnBase  CompositeWrenchFrame=BaseFrame  SenseConstraintForce=off  SenseConstraintTorque=off  SenseTotalForce=off  SenseTotalTorque=off  PositionTargetSpecify=on  PositionTargetPriority=Low  PositionTargetValue=initChassisToBoomRevPos  PositionTargetValueUnits=deg  VelocityTargetSpecify=off  VelocityTargetPriority=High  VelocityTargetValue=0  VelocityTargetValueUnits=deg/s  EquilibriumPosition=0  EquilibriumPositionUnits=deg  SpringStiffness=0  SpringStiffnessUnits=N*m/deg  DampingCoefficient=0  DampingCoefficientUnits=N*m/(deg/s)  LowerLimitSpecify=off  LowerLimitBound=-90  LowerLimitBoundUnits=deg  LowerLimitStiffness=1e4  LowerLimitStiffnessUnits=N*m/deg  LowerLimitDamping=10  LowerLimitDampingUnits=N*m/(deg/s)  LowerLimitTransitionRegionWidth=0.1  LowerLimitTransitionRegionWidthUnits=deg  UpperLimitSpecify=off  UpperLimitBound=90  UpperLimitBoundUnits=deg  UpperLimitStiffness=1e4  UpperLimitStiffnessUnits=N*m/deg  UpperLimitDamping=10  UpperLimitDampingUnits=N*m/(deg/s)  UpperLimitTransitionRegionWidth=0.1  UpperLimitTransitionRegionWidthUnits=deg  TorqueActuationMode=NoTorque  MotionActuationMode=ComputedMotion  SensePosition=off  SenseVelocity=off  SenseAcceleration=off  SenseTorqueForce=off  SenseLowerLimitTorqueForce=off  SenseUpperLimitTorqueForce=off
  Connection Label : ConnectionLabel  Label=Cha
  Connection Label1 : ConnectionLabel  Label=Cha
  Gravity : Subsystem
  Ground : Subsystem
      mask Display: image('DesolateOutbackProjectionTarget.png');
  Ground Contact : Subsystem
  Label B1 : ConnectionLabel  Label=B
  Label B2 : ConnectionLabel  Label=B
  Mechanism Configuration : sm_lib/Utilities/Mechanism Configuration  UniformGravity=TimeVarying  GravityVector=[0 0 -9.80665]  GravityVectorUnits=m/s^2  LinearizationDelta=0.001  JointModeTransitionNonlinearIterations=2
  Mevea : Subsystem
      mask Display: image('MEVEA_Icon.jpg')
  Pos CG : Subsystem
  Simulink-PS Converter : nesl_utility/Simulink-PS Converter  PhysicalDomain=network_engine_domain  SubClassName=ps_input  LeftPortType=input  RightPortType=output  PseudoPeriodic=off  Frequencies=[]  NoiseDistribution=none  NoiseParameters=[]  Unit=m/s^2  AffineConversion=off  FilteringAndDerivatives=provide  SimscapeFilterOrder=1  InputFilterTimeConstant=0.001  UdotUserProvided=0
  Stick : Excavator_Parts_Lib/Stick  Tag=62A93771-C790-5E4F-BFD2-96C4D317E04B  opc=1  part_clr=excv_data.arm.clr
  Stick Cyl : Subsystem
      mask Display: image('Excavator_Cylinder_Actuate_IMAGE.png')
  StickToBucket : Subsystem  Tag=07adba86-714b-4e09-8ef8-8682a71cd5e3
      mask Display: image('Excavator_Revolute_IMAGE.png')
  World Frame : sm_lib/Frames and Transforms/World Frame
  fNormal : Scope  NumInputPorts=2
      settings: ActiveDisplayYMinimum=-49246.03186  ActiveDisplayYMaximum=443214.28677  DataLoggingVariableName=ScopeData4
  StickCyl : PMIOPort  Side=Left
  BucketCyl : PMIOPort  Port=2  Side=Left
  BoomHyd : PMIOPort  Port=3  Side=Left
  SwingMotor : PMIOPort  Port=4  Side=Left
  SwingSpeed : Outport
  wires:
  BaseToChassis/1(m) -> SwingSpeed/1
  Gravity/1(g) -> Simulink-PS Converter/1
  Ground Contact/1(m) -> Bus Selector/1
  Bus Selector/1 -> fNormal/1  "<fn>"
  Bus Selector/2 -> fNormal/2  "<ff>"
  connections:
  Chassis/LConn1 -- Connection Label/LConn1 -- BaseToChassis/RConn1
  Base/RConn1 -- BaseToChassis/LConn2
  SwingMotor/RConn1 -- BaseToChassis/LConn1
  Chassis/RConn2 -- ChassisToBoom/LConn1
  Boom/RConn3 -- Boom ToStick/LConn1
  Stick/RConn5 -- StickToBucket/LConn1
  Stick/RConn2 -- Bucket Cyl/LConn2
  Stick/RConn4 -- Bucket Linkage/LConn1
  Stick/RConn3 -- Bucket Linkage/LConn2
  Simulink-PS Converter/RConn1 -- Mechanism Configuration/LConn1
  Mechanism Configuration/RConn1 -- World Frame/RConn1 -- 6-DOF Joint/LConn1 -- Ground Contact/LConn1 -- Ground/RConn1
  Base/LConn1 -- Ground Contact/RConn1 -- 6-DOF Joint/RConn1
  Boom/LConn1 -- ChassisToBoom/RConn1
  Boom/RConn2 -- Stick Cyl/LConn2
  Bucket/LConn2 -- BucketLink ToBucket/RConn1
  Bucket Linkage/RConn1 -- BucketLink ToBucket/LConn1
  Pos CG/RConn1 -- Bucket/RConn2
  Boom/RConn1 -- Boom Cyl L/RConn2
  Label B1/LConn1 -- Boom Cyl L/LConn1
  Chassis/RConn1 -- Boom Cyl L/LConn2
  Chassis/RConn3 -- Boom Cyl R/LConn2
  Boom/RConn4 -- Boom Cyl R/RConn2
  BoomHyd/RConn1 -- B/LConn1
  Label B2/LConn1 -- Boom Cyl R/LConn1
  StickCyl/RConn1 -- Stick Cyl/LConn1
  Stick/RConn1 -- Stick Cyl/RConn2
  Stick/LConn1 -- Boom ToStick/RConn1
  Bucket Linkage/LConn3 -- Bucket Cyl/RConn2
  BucketCyl/RConn1 -- Bucket Cyl/LConn1
  Pos CG/LConn1 -- Connection Label1/LConn1
  StickToBucket/RConn1 -- Bucket/LConn1 -- Mevea/RConn1

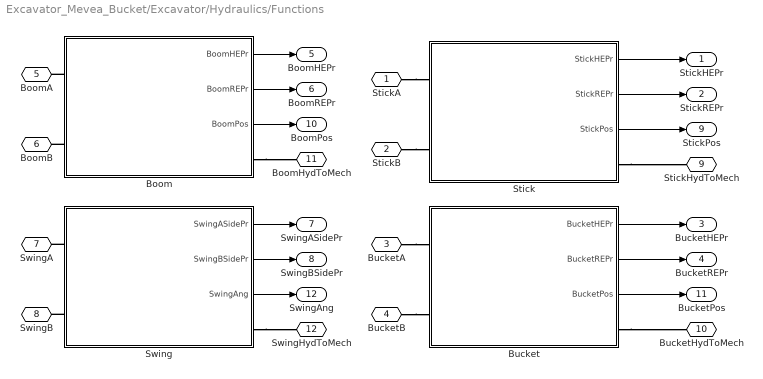
== system Excavator_Mevea_Bucket/Excavator/Hydraulics/Functions ==
  Boom : Subsystem
      mask Display: image('Actuator_2Cyl_IMAGE.png')
  Bucket : Subsystem
      mask Display: image('Actuator_1Cyl_IMAGE.png');
  Stick : Subsystem
      mask Display: image('Actuator_1Cyl_IMAGE.png');
  Swing : Subsystem
      mask Display: image('Actuator_1Motor_IMAGE.png');
  StickA : PMIOPort  Side=Left
  StickB : PMIOPort  Port=2  Side=Left
  BucketA : PMIOPort  Port=3  Side=Left
  BucketB : PMIOPort  Port=4  Side=Left
  BoomA : PMIOPort  Port=5  Side=Left
  BoomB : PMIOPort  Port=6  Side=Left
  SwingA : PMIOPort  Port=7  Side=Left
  SwingB : PMIOPort  Port=8  Side=Left
  StickHydToMech : PMIOPort  Port=9  Side=Right
  BucketHydToMech : PMIOPort  Port=10  Side=Right
  BoomHydToMech : PMIOPort  Port=11  Side=Right
  SwingHydToMech : PMIOPort  Port=12  Side=Right
  StickHEPr : Outport
  StickREPr : Outport  Port=2
  BucketHEPr : Outport  Port=3
  BucketREPr : Outport  Port=4
  BoomHEPr : Outport  Port=5
  BoomREPr : Outport  Port=6
  SwingASidePr : Outport  Port=7
  SwingBSidePr : Outport  Port=8
  StickPos : Outport  Port=9
  BoomPos : Outport  Port=10
  BucketPos : Outport  Port=11
  SwingAng : Outport  Port=12
  wires:
  Stick/2(StickREPr) -> StickREPr/1
  Stick/1(StickHEPr) -> StickHEPr/1
  Bucket/2(BucketREPr) -> BucketREPr/1
  Bucket/1(BucketHEPr) -> BucketHEPr/1
  Boom/2(BoomREPr) -> BoomREPr/1
  Boom/1(BoomHEPr) -> BoomHEPr/1
  Swing/2(SwingBSidePr) -> SwingBSidePr/1
  Swing/1(SwingASidePr) -> SwingASidePr/1
  Stick/3(StickPos) -> StickPos/1
  Boom/3(BoomPos) -> BoomPos/1
  Bucket/3(BucketPos) -> BucketPos/1
  Swing/3(SwingAng) -> SwingAng/1
  connections:
  Swing/LConn2 -- SwingB/RConn1
  Swing/RConn1 -- SwingHydToMech/RConn1
  BucketA/RConn1 -- Bucket/LConn1
  StickA/RConn1 -- Stick/LConn1
  BucketB/RConn1 -- Bucket/LConn2
  Boom/RConn1 -- BoomHydToMech/RConn1
  StickB/RConn1 -- Stick/LConn2
  Boom/LConn2 -- BoomB/RConn1
  Stick/RConn1 -- StickHydToMech/RConn1
  Bucket/RConn1 -- BucketHydToMech/RConn1
  Boom/LConn1 -- BoomA/RConn1
  Swing/LConn1 -- SwingA/RConn1

== system Excavator_Mevea_Bucket/Excavator/Hydraulics/LeftPump ==
  Cmd : Inport
  LeftPump : SimscapeFluids_lib/Isothermal Liquid/Pumps & Motors/Variable-Displacement Pump (IL)  leakage_friction_spec=fluids.isothermal_liquid.pumps_motors.enum.pump_motor_loss_spec.input_efficiency  displacement_nominal=30 cm^3/rev  omega_nominal=188 rad/s  p_nominal=10 MPa  vol_eff_nominal=0.92  mech_eff_nominal=0.88  no_load_torque=0 N*m  p_diff_eff_TLU=[.1, 1, 2] MPa  omega_eff_TLU=[25, 50, 100, 200, 300, 400] rad/s  displacement_eff_TLU=[-30, -19, 19, 30] cm^3/rev  vol_eff_TLU=repmat([.816, .908, .954, .977, .981, .984; .325, .663, .831, .916, .925, .946; .137, .568, .78, .892, .893, .91], 1, 1, 4)  mech_eff_TLU=repmat([.996, .996, .996, .996, .996, .996; .988, .989, .989, .989, .989, .99; .981, .981, .982, .982, .983, .984], 1, 1, 4)  p_diff_loss_TLU=[.1, 1, 2] MPa  omega_loss_TLU=[25, 50, 100, 200, 300, 400] rad/s  displacement_loss_TLU=[-30, -19, 19, 30] cm^3/rev  vol_loss_TLU=repmat(1e-3 * [.023, .023, .023, .023, .0285, .032; .0844, .0842, .0845, .084, .1125, .108; .1079, .108, .11, .108, .1605, .18], 1, 1, 4) m^3/s  mech_loss_TLU=repmat([.002, .002, .002, .002, .002, .002; .0607, .0556, .0556, .0556, .0556, .0505; .1937, .1937, .1833, .1833, .1729, .1626], 1, 1, 4) N*m  vol_eff_min=1e-3  vol_eff_max=1  mech_eff_min=1e-3  mech_eff_max=1  pressure_threshold=1e-3 MPa  omega_threshold=10 rad/s  displacement_threshold=0.1 cm^3/rev  supplied_range_check=simscape.enum.assert.action.none  pump_mode_check=simscape.enum.assert.action.none  pressure_check=simscape.enum.assert.action.none  p_min_valid=0.101325 MPa
  LeftPumpEM : fl_lib/Physical Signals/Sources/PS Constant  constant=1
  LeftPumpEV : fl_lib/Physical Signals/Sources/PS Constant  constant=1
  LeftPumpPrSensor : fl_lib/Isothermal Liquid/Sensors/Pressure Sensor (IL)  pressure_measure=foundation.enum.pressure_measure.gauge
  LeftPumpVolChamber : fl_lib/Isothermal Liquid/Elements/Constant Volume Chamber (IL)  volume=pumpChamberVol mm^3  p_I_specify=on  p_I_priority=High  p_I=p0 bar  p_I_nominal_specify=off  p_I_nominal_value=1  p_I_nominal_unit=MPa
  Mechanical Rotational Reference : fl_lib/Mechanical/Rotational Elements/Mechanical Rotational Reference
  PS-Simulink Converter1 : nesl_utility/PS-Simulink Converter  PhysicalDomain=network_engine_domain  SubClassName=ps_output  LeftPortType=input  RightPortType=output  PseudoPeriodic=off  Frequencies=[]  VectorFormat=1-D array  Unit=bar  AffineConversion=off
  Simulink-PS Converter2 : nesl_utility/Simulink-PS Converter  PhysicalDomain=network_engine_domain  SubClassName=ps_input  LeftPortType=input  RightPortType=output  PseudoPeriodic=off  Frequencies=[]  NoiseDistribution=none  NoiseParameters=[]  Unit=cm^3/rev  AffineConversion=off  FilteringAndDerivatives=provide  SimscapeFilterOrder=1  InputFilterTimeConstant=0.01  UdotUserProvided=0
  Transfer Fcn (with initial outputs) : simulink_extras/Additional Linear/Transfer Fcn (with initial outputs)  N=[1]  D="[0.01  1]"  Y0=p0  U0=p0
  R : PMIOPort  Side=Left
  A : PMIOPort  Port=2  Side=Left
  B : PMIOPort  Port=3  Side=Right
  p : Outport
  wires:
  PS-Simulink Converter1/1 -> Transfer Fcn (with initial outputs)/1
  Transfer Fcn (with initial outputs)/1 -> p/1
  Cmd/1 -> Simulink-PS Converter2/1
  connections:
  Simulink-PS Converter2/RConn1 -- LeftPump/LConn1
  LeftPumpPrSensor/RConn1 -- PS-Simulink Converter1/LConn1
  LeftPump/LConn4 -- B/RConn1 -- LeftPumpPrSensor/LConn1 -- LeftPumpVolChamber/LConn1
  LeftPump/RConn2 -- Mechanical Rotational Reference/LConn1
  LeftPump/LConn2 -- LeftPumpEV/RConn1
  LeftPump/LConn3 -- LeftPumpEM/RConn1
  LeftPump/RConn3 -- A/RConn1
  LeftPump/RConn1 -- R/RConn1
